simulink model "ad9361_rx_wlan_testbench_targeting_org"  (Simulink 10.0)
settings: Solver=FixedStepDiscrete  StartTime=0.0  StopTime=2  RelTol=1e-3
InitFcn:
  | % General
  | FFT = 64;
  | LSTFSymbol = FFT/4;
  | FS = 20e6;
  | 
  | % NCO
  | Fs = 20e6;
  | res = 0.05;
  | SFDR = 100;
  | N = ceil(log2(Fs/res));
  | %trueRes = Fs/(2^N);
  | %phaseInc = round(Fc*2^N/Fs);
  | QAB = round((SFDR-12)/6);
  | Dither = N - QAB;
  | 
  | %% LLTF
  | a = load('lltf.mat');
  | lltfFlip = conj(flipud(a.LLTF(:, 1)));
  | 
  | lltfFlip = lltfFlip./(max(abs(lltfFlip))) .* 2^0;
libraries: simulink x9, dsphdlfiltering x5, hdlsllib x4, commsource2 x1, dspmathops x1, dspsigops x1
(part 1 of 2)
settings Model: DataTypeOverride=Off  Creator=tcollins  LastModifiedBy=bhisma  SimulationMode=accelerator
settings Model: SuppressorTable=|
  | <?xml version="1.0" encoding="UTF-8" standalone="yes" ?>
  | <!DOCTYPE boost_serialization>
  | <boost_serialization signature="serialization::archive" version="15">
  | <DiagnosticSuppressor class_id="0" tracking_level="0" version="6">
  | 	<Table class_id="1" tracking_level="0" version="0">
  | 		<count>4</count>
  | 		<bucket_count>5</bucket_count>
  | 		<item_version>0</item_version>
  | 		<item class_id="2" tracking_level="0" version="0">
  | 			<first class_id="3" tracking_level="0" version="6">
  | 				<Source class_id="4" tracking_level="0" version="0">
  | 					<count>1</count>
  | 					<item_version>0</item_version>
  | 					<item>ad9361_rx_wlan_testbench_targeting_org/HDL_DUT/Control AGC/HDL Counter</item>
  | 				</Source>
  | 			</first>
  | 			<second class_id="5" tracking_level="0" version="6">
  | 				<SuppressedData class_id="6" tracking_level="0" version="0">
  | 					<count>2</count>
  | 					<bucket_count>2</bucket_count>
  | 					<item_version>0</item_version>
  | 					<item class_id="7" tracking_level="0" version="0">
  | 						<first class_id="8" tracking_level="0" version="6">
  | 							<ID>SimulinkFixedPoint:util:Overflowoccurred</ID>
  | 							<Cause>
  | 								<Source>
  | 									<count>0</count>
  | 									<item_version>0</item_version>
  | 								</Source>
  | 							</Cause>
  | 						</first>
  | 						<second class_id="9" tracking_level="0" version="6">
  | 							<Comment></Comment>
  | 							<User></User>
  | 							<LastModified class_id="10" tracking_level="0" version="0">
  | 								<ptime_date class_id="11" tracking_level="0" version="0">
  | 									<date>20160715</date>
  | 								</ptime_date>
  | 								<ptime_time_duration class_id="12" tracking_level="0" version="0">
  | 									<is_special>0</is_special>
  | 									<time_duration_hours>14</time_duration_hours>
  | 									<time_duration_minutes>21</time_duration_minutes>
  | 									<time_duration_seconds>36</time_duration_seconds>
  | 									<time_duration_fractional_seconds>0</time_duration_fractional_seconds>
  | 								</ptime_time_duration>
  | 							</LastModified>
  | 							<SuppressionType>1</SuppressionType>
  | 						</second>
  | 					</item>
  | 					<item>
  | 						<first>
  | 							<ID>Simulink:DataType:WarningOverFlowDetected</ID>
  | 							<Cause>
  | 								<Source>
  | 									<count>0</count>
  | 									<item_version>0</item_version>
  | 								</Source>
  | 							</Cause>
  | 						</first>
  | 						<second>
  | 							<Comment></Comment>
  | 							<User></User>
  | 							<LastModified>
  | 								<ptime_date>
  | 									<date>20160715</date>
  | 								</ptime_date>
  | 								<ptime_time_duration>
  | 									<is_special>0</is_special>
  | 									<time_duration_hours>14</time_duration_hours>
  | 									<time_duration_minutes>21</time_duration_minutes>
  | 									<time_duration_seconds>36</time_duration_seconds>
  | 									<time_duration_fractional_seconds>0</time_duration_fractional_seconds>
  | 								</ptime_time_duration>
  | 							</LastModified>
  | 							<SuppressionType>1</SuppressionType>
  | 						</second>
  | 					</item>
  | 				</SuppressedData>
  | 			</second>
  | 		</item>
  | 		<item>
  | 			<first>
  | 				<Source>
  | 					<count>1</count>
  | 					<item_version>0</item_version>
  | 					<item>ad9361_rx_wlan_testbench_targeting_org/HDL_DUT/Debug/HDL Counter3</item>
  | 				</Source>
  | 			</first>
  | 			<second>
  | 				<SuppressedData>
  | 					<count>2</count>
  | 					<bucket_count>2</bucket_count>
  | 					<item_version>0</item_version>
  | 					<item>
  | 						<first>
  | 							<ID>Simulink:DataType:WarningOverFlowDetected</ID>
  | 							<Cause>
  | 								<Source>
  | 									<count>0</count>
  | 									<item_version>0</item_version>
  | 								</Source>
  | 							</Cause>
  | 						</first>
  | 						<second>
  | 							<Comment></Comment>
  | 							<User></User>
  | 							<LastModified>
  | 								<ptime_date>
  | 									<date>20160715</date>
  | 								</ptime_date>
  | 								<ptime_time_duration>
  | 									<is_special>0</is_special>
  | 									<time_duration_hours>14</time_duration_hours>
  | 									<time_duration_minutes>21</time_duration_minutes>
  | 									<time_duration_seconds>36</time_duration_seconds>
  | 									<time_duration_fractional_seconds>0</time_duration_fractional_seconds>
  | 								</ptime_time_duration>
  | 							</LastModified>
  | 							<SuppressionType>1</SuppressionType>
  | 						</second>
  | 					</item>
  | 					<item>
  | 						<first>
  | 							<ID>SimulinkFixedPoint:util:Overflowoccurred</ID>
  | 							<Cause>
  | 								<Source>
  | 									<count>0</count>
  | 									<item_version>0</item_version>
  | 								</Source>
  | 							</Cause>
  | 						</first>
  | 						<second>
  | 							<Comment></Comment>
  | 							<User></User>
  | 							<LastModified>
  | 								<ptime_date>
  | 									<date>20160715</date>
  | 								</ptime_date>
  | 								<ptime_time_duration>
  | 									<is_special>0</is_special>
  | 									<time_duration_hours>14</time_duration_hours>
  | 									<time_duration_minutes>21</time_duration_minutes>
  | 									<time_duration_seconds>36</time_duration_seconds>
  | 									<time_duration_fractional_seconds>0</time_duration_fractional_seconds>
  | 								</ptime_time_duration>
  | 							</LastModified>
  | 							<SuppressionType>1</SuppressionType>
  | 						</second>
  | 					</item>
  | 				</SuppressedData>
  | 			</second>
  | 		</item>
  | 		<item>
  | 			<first>
  | 				<Source>
  | 					<count>1</count>
  | 					<item_version>0</item_version>
  | 					<item>ad9361_rx_wlan_testbench_targeting_org/HDL_DUT/Debug/HDL Counter2</item>
  | 				</Source>
  | 			</first>
  | 			<second>
  | 				<SuppressedData>
  | 					<count>2</count>
  | 					<bucket_count>2</bucket_count>
  | 					<item_version>0</item_version>
  | 					<item>
  | 						<first>
  | 							<ID>Simulink:DataType:WarningOverFlowDetected</ID>
  | 							<Cause>
  | 								<Source>
  | 									<count>0</count>
  | 									<item_version>0</item_version>
  | 								</Source>
  | 							</Cause>
  | 						</first>
  | 						<second>
  | 							<Comment></Comment>
  | 							<User></User>
  | 							<LastModified>
  | 								<ptime_date>
  | 									<date>20160715</date>
  | 								</ptime_date>
  | 								<ptime_time_duration>
  | 									<is_special>0</is_special>
  | 									<time_duration_hours>14</time_duration_hours>
  | 									<time_duration_minutes>21</time_duration_minutes>
  | 									<time_duration_seconds>36</time_duration_seconds>
  | 									<time_duration_fractional_seconds>0</time_duration_fractional_seconds>
  | 								</ptime_time_duration>
  | 							</LastModified>
  | 							<SuppressionType>1</SuppressionType>
  | 						</second>
  | 					</item>
  | 					<item>
  | 						<first>
  | 							<ID>SimulinkFixedPoint:util:Overflowoccurred</ID>
  | 							<Cause>
  | 								<Source>
  | 									<count>0</count>
  | 									<item_version>0</item_version>
  | 								</Source>
  | 							</Cause>
  | 						</first>
  | 						<second>
  | 							<Comment></Comment>
  | 							<User></User>
  | 							<LastModified>
  | 								<ptime_date>
  | 									<date>20160715</date>
  | 								</ptime_date>
  | 								<ptime_time_duration>
  | 									<is_special>0</is_special>
  | 									<time_duration_hours>14</time_duration_hours>
  | 									<time_duration_minutes>21</time_duration_minutes>
  | 									<time_duration_seconds>36</time_duration_seconds>
  | 									<time_duration_fractional_seconds>0</time_duration_fractional_seconds>
  | 								</ptime_time_duration>
  | 							</LastModified>
  | 							<SuppressionType>1</SuppressionType>
  | 						</second>
  | 					</item>
  | 				</SuppressedData>
  | 			</second>
  | 		</item>
  | 		<item>
  | 			<first>
  | 				<Source>
  | 					<count>1</count>
  | 					<item_version>0</item_version>
  | 					<item>ad9361_rx_wlan_testbench_targeting_org/HDL_DUT/Debug/HDL Counter1</item>
  | 				</Source>
  | 			</first>
  | 			<second>
  | 				<SuppressedData>
  | 					<count>2</count>
  | 					<bucket_count>2</bucket_count>
  | 					<item_version>0</item_version>
  | 					<item>
  | 						<first>
  | 							<ID>Simulink:DataType:WarningOverFlowDetected</ID>
  | 							<Cause>
  | 								<Source>
  | 									<count>0</count>
  | 									<item_version>0</item_version>
  | 								</Source>
  | 							</Cause>
  | 						</first>
  | 						<second>
  | 							<Comment></Comment>
  | 							<User></User>
  | 							<LastModified>
  | 								<ptime_date>
  | 									<date>20160715</date>
  | 								</ptime_date>
  | 								<ptime_time_duration>
  | 									<is_special>0</is_special>
  | 									<time_duration_hours>14</time_duration_hours>
  | 									<time_duration_minutes>21</time_duration_minutes>
  | 									<time_duration_seconds>36</time_duration_seconds>
  | 									<time_duration_fractional_seconds>0</time_duration_fractional_seconds>
  | 								</ptime_time_duration>
  | 							</LastModified>
  | 							<SuppressionType>1</SuppressionType>
  | 						</second>
  | 					</item>
  | 					<item>
  | 						<first>
  | 							<ID>SimulinkFixedPoint:util:Overflowoccurred</ID>
  | 							<Cause>
  | 								<Source>
  | 									<count>0</count>
  | 									<item_version>0</item_version>
  | 								</Source>
  | 							</Cause>
  | 						</first>
  | 						<second>
  | 							<Comment></Comment>
  | 							<User></User>
  | 							<LastModified>
  | 								<ptime_date>
  | 									<date>20160715</date>
  | 								</ptime_date>
  | 								<ptime_time_duration>
  | 									<is_special>0</is_special>
  | 									<time_duration_hours>14</time_duration_hours>
  | 									<time_duration_minutes>21</time_duration_minutes>
  | 									<time_duration_seconds>36</time_duration_seconds>
  | 									<time_duration_fractional_seconds>0</time_duration_fractional_seconds>
  | 								</ptime_time_duration>
  | 							</LastModified>
  | 							<SuppressionType>1</SuppressionType>
  | 						</second>
  | 					</item>
  | 				</SuppressedData>
  | 			</second>
  | 		</item>
  | 	</Table>
  | </DiagnosticSuppressor>
  | </boost_serialization>
settings DataIOCC: LimitDataPoints=on  SaveFormat=Dataset  SaveOutput=off  SaveTime=off
settings OptimizationCC: BlockReduction=off  ConditionallyExecuteInputs=off  DefaultParameterBehavior=Inlined
settings DebuggingCC: SignalRangeChecking=error  AlgebraicLoopMsg=error  UnderspecifiedInitializationDetection=Simplified  MergeDetectMultiDrivingBlocksExec=error  SingleTaskRateTransMsg=error  IntegerOverflowMsg=none  ParameterDowncastMsg=none  ParameterOverflowMsg=none  ParameterPrecisionLossMsg=none  AllowSymbolicDim=off  StrictBusMsg=ErrorOnBusTreatedAsVector  IntegerSaturationMsg=none
settings HardwareCC: ProdHWDeviceType=ASIC/FPGA->ASIC/FPGA  ProdEqTarget=off
settings ModelReferenceCC: PropagateSignalLabelsOutOfModel=on
settings GRTTargetCC: GeneratePreprocessorConditionals=Disable all  CombineOutputUpdateFcns=on  GRTInterface=off
settings ConfigComp: CovScope=ReferencedModels  CovExternalEMLEnable=off  CovSFcnEnable=off

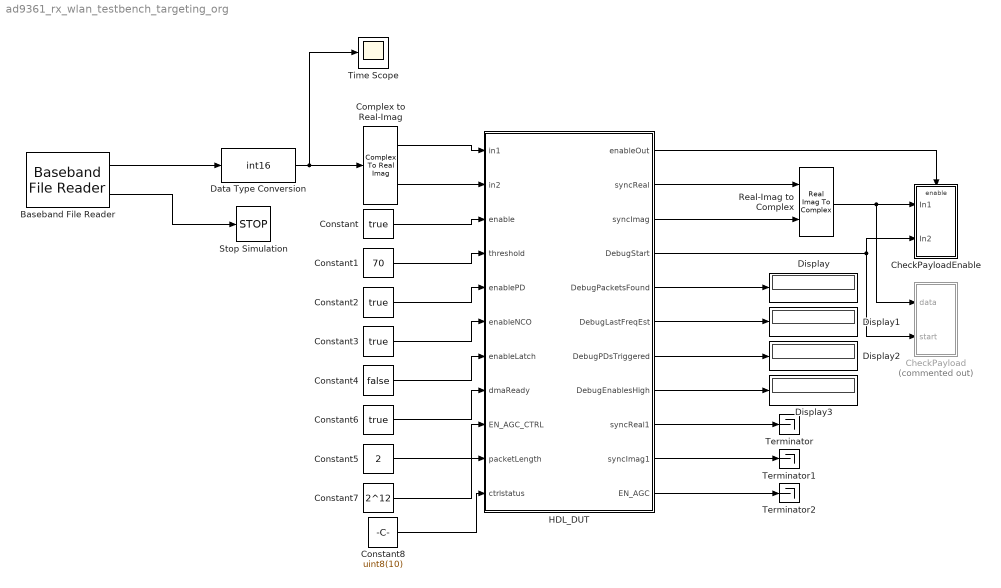
== system ad9361_rx_wlan_testbench_targeting_org ==
  Baseband File Reader : commsource2/Baseband File Reader  Filename=./captures/IQData_m25.bb  InheritSampleTimeFromFile=on  SampleTime=1  SamplesPerFrame=1  CyclicRepetition=off  FileEndOutputPort=on  SimulateUsing=Interpreted execution
      settings: SourceProductName=Communications Toolbox  SourceProductBaseCode=CM
  CheckPayload : Subsystem  Commented=on
  CheckPayloadEnable : Subsystem
  Complex to Real-Imag : ComplexToRealImag
  Constant{,2..3,6} (4 alike) : Constant  Value=true  SampleTime=-1
  Constant1 : Constant  Value=70  OutDataTypeStr=int16  SampleTime=-1
  Constant4 : Constant  Value=false  SampleTime=-1  LockScale=on
  Constant5 : Constant  Value=2  OutDataTypeStr=uint32  SampleTime=-1  LockScale=on
  Constant7 : Constant  Value=2^12  OutDataTypeStr=uint32  SampleTime=-1  LockScale=on
  Constant8 : Constant  Value=uint8(10)  OutDataTypeStr=uint8  SampleTime=-1  LockScale=on
  Data Type Conversion : DataTypeConversion  OutDataTypeStr=int16
  Display{,1..3} (4 alike) : Display
  HDL_DUT : Subsystem  TreatAsAtomicUnit=on
  Real-Imag to Complex : RealImagToComplex
  Stop Simulation : Stop
  Terminator : Terminator
  Terminator1 : Terminator
  Terminator2 : Terminator
  Time Scope : Scope
  wires:
  Constant/1 -> HDL_DUT/3(enable)
  Complex to Real-Imag/1 -> HDL_DUT/1(in1)
  Complex to Real-Imag/2 -> HDL_DUT/2(in2)
  Baseband File Reader/1 -> Data Type Conversion/1
  Constant1/1 -> HDL_DUT/4(threshold)
  Constant2/1 -> HDL_DUT/5(enablePD)
  Constant3/1 -> HDL_DUT/6(enableNCO)
  HDL_DUT/7(DebugPDsTriggered) -> Display2/1
  HDL_DUT/5(DebugPacketsFound) -> Display/1
  Real-Imag to Complex/1 -> CheckPayload/1(data), CheckPayloadEnable/1(In1)
  HDL_DUT/4(DebugStart) -> CheckPayloadEnable/2(In2), CheckPayload/2(start)
  HDL_DUT/6(DebugLastFreqEst) -> Display1/1
  HDL_DUT/8(DebugEnablesHigh) -> Display3/1
  HDL_DUT/2(syncReal) -> Real-Imag to Complex/1
  HDL_DUT/3(syncImag) -> Real-Imag to Complex/2
  HDL_DUT/1(enableOut) -> CheckPayloadEnable/Enable
  Data Type Conversion/1 -> Time Scope/1, Complex to Real-Imag/1
  HDL_DUT/9(syncReal1) -> Terminator/1
  HDL_DUT/10(syncImag1) -> Terminator1/1
  Constant4/1 -> HDL_DUT/7(enableLatch)
  Constant5/1 -> HDL_DUT/9(EN_AGC_CTRL)
  Constant6/1 -> HDL_DUT/8(dmaReady)
  Constant7/1 -> HDL_DUT/10(packetLength)
  HDL_DUT/11(EN_AGC) -> Terminator2/1
  Baseband File Reader/2 -> Stop Simulation/1
  Constant8/1 -> HDL_DUT/11(ctrlstatus)

== system ad9361_rx_wlan_testbench_targeting_org/CheckPayload ==
  data : Inport  OutDataTypeStr=int16
  start : Inport  Port=2
  Check LSIG1 : MATLAB Function  TreatAsAtomicUnit=on
  SaveData : Subsystem
  wires:
  Check LSIG1/2(goodPackets) -> SaveData/1(In1)
  start/1 -> Check LSIG1/1(start)
  Check LSIG1/1(valid) -> SaveData/Enable
  data/1 -> Check LSIG1/2(data)
  Check LSIG1/3(badPackets) -> SaveData/2(In2)

== system ad9361_rx_wlan_testbench_targeting_org/CheckPayloadEnable ==
  In1 : Inport
  In2 : Inport  Port=2
  Enable : EnablePort
  Check LSIG1 : MATLAB Function  TreatAsAtomicUnit=on
  SaveData : Subsystem
  wires:
  Check LSIG1/2(goodPackets) -> SaveData/1(In1)
  Check LSIG1/1(valid) -> SaveData/Enable
  In1/1 -> Check LSIG1/2(data)
  Check LSIG1/3(badPackets) -> SaveData/2(In2)
  In2/1 -> Check LSIG1/1(start)

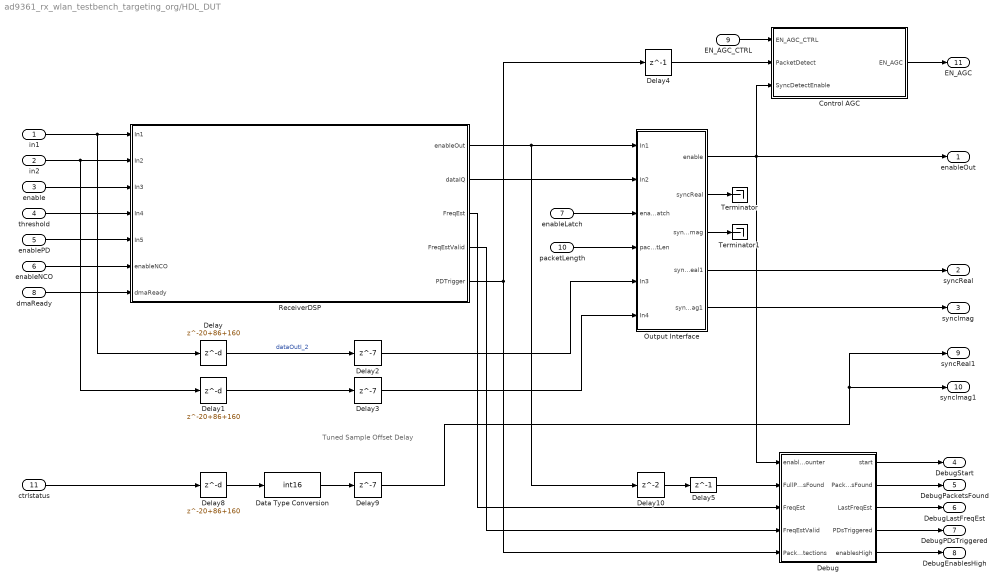
== system ad9361_rx_wlan_testbench_targeting_org/HDL_DUT ==
  note: Tuned Sample Offset Delay
  in1 : Inport  OutDataTypeStr=int16
  in2 : Inport  Port=2  OutDataTypeStr=int16
  enable : Inport  Port=3  OutDataTypeStr=boolean  LockScale=on
  threshold : Inport  Port=4  OutDataTypeStr=int16  LockScale=on
  enablePD : Inport  Port=5  OutDataTypeStr=boolean  LockScale=on
  enableNCO : Inport  Port=6  OutDataTypeStr=boolean  LockScale=on
  enableLatch : Inport  Port=7  OutDataTypeStr=boolean  LockScale=on
  dmaReady : Inport  Port=8  OutDataTypeStr=boolean
  EN_AGC_CTRL : Inport  Port=9  OutDataTypeStr=uint32
  packetLength : Inport  Port=10  OutDataTypeStr=uint32  LockScale=on
  ctrlstatus : Inport  Port=11  OutDataTypeStr=uint8
  Control AGC : Subsystem
  Data Type Conversion : DataTypeConversion  OutDataTypeStr=int16
  Debug : Subsystem
  Delay : Delay  DelayLength=20+86+160
  Delay1 : Delay  DelayLength=20+86+160
  Delay10 : Delay
  Delay2 : Delay  DelayLength=7
  Delay3 : Delay  DelayLength=7
  Delay4 : Delay  DelayLength=1
  Delay5 : Delay  DelayLength=1
  Delay8 : Delay  DelayLength=20+86+160
  Delay9 : Delay  DelayLength=7
  Output Interface : Subsystem
  ReceiverDSP : Subsystem
  Terminator : Terminator
  Terminator1 : Terminator
  enableOut : Outport  VectorParamsAs1DForOutWhenUnconnected=off
  syncReal : Outport  Port=2  OutDataTypeStr=int16  VectorParamsAs1DForOutWhenUnconnected=off
  syncImag : Outport  Port=3  OutDataTypeStr=int16  VectorParamsAs1DForOutWhenUnconnected=off
  DebugStart : Outport  Port=4  VectorParamsAs1DForOutWhenUnconnected=off
  DebugPacketsFound : Outport  Port=5  VectorParamsAs1DForOutWhenUnconnected=off
  DebugLastFreqEst : Outport  Port=6  VectorParamsAs1DForOutWhenUnconnected=off
  DebugPDsTriggered : Outport  Port=7  VectorParamsAs1DForOutWhenUnconnected=off
  DebugEnablesHigh : Outport  Port=8  VectorParamsAs1DForOutWhenUnconnected=off
  syncReal1 : Outport  Port=9  OutDataTypeStr=int16  VectorParamsAs1DForOutWhenUnconnected=off
  syncImag1 : Outport  Port=10  OutDataTypeStr=int16  VectorParamsAs1DForOutWhenUnconnected=off
  EN_AGC : Outport  Port=11  OutDataTypeStr=boolean  VectorParamsAs1DForOutWhenUnconnected=off
  wires:
  Debug/2(PacketsFound) -> DebugPacketsFound/1
  Debug/3(LastFreqEst) -> DebugLastFreqEst/1
  Debug/5(enablesHigh) -> DebugEnablesHigh/1
  Debug/4(PDsTriggered) -> DebugPDsTriggered/1
  Debug/1(start) -> DebugStart/1
  Output Interface/1(enable) -> enableOut/1, Control AGC/3(SyncDetectEnable), Debug/1(enableCounter)
  ReceiverDSP/1(enableOut) -> Output Interface/1(In1), Delay10/1
  in2/1 -> Delay1/1, ReceiverDSP/2(In2)
  enable/1 -> ReceiverDSP/3(In3)
  threshold/1 -> ReceiverDSP/4(In4)
  enablePD/1 -> ReceiverDSP/5(In5)
  enableNCO/1 -> ReceiverDSP/6(enableNCO)
  ReceiverDSP/3(FreqEst) -> Debug/3(FreqEst)
  ReceiverDSP/4(FreqEstValid) -> Debug/4(FreqEstValid)
  ReceiverDSP/5(PDTrigger) -> Delay4/1, Debug/5(PacketDetections)
  in1/1 -> Delay/1, ReceiverDSP/1(In1)
  Delay/1 -> Delay2/1  "dataOutI_2"
  enableLatch/1 -> Output Interface/3(enableLatch)
  Control AGC/1(EN_AGC) -> EN_AGC/1
  EN_AGC_CTRL/1 -> Control AGC/1(EN_AGC_CTRL)
  dmaReady/1 -> ReceiverDSP/7(dmaReady)
  Output Interface/2(syncReal) -> Terminator/1
  Output Interface/3(syncImag) -> Terminator1/1
  Delay1/1 -> Delay3/1
  packetLength/1 -> Output Interface/4(packetLen)
  Delay4/1 -> Control AGC/2(PacketDetect)
  Delay5/1 -> Debug/2(FullPacketsFound)
  ReceiverDSP/2(dataIQ) -> Output Interface/2(In2)
  Delay10/1 -> Delay5/1
  Output Interface/4(syncReal1) -> syncReal/1
  Output Interface/5(syncImag1) -> syncImag/1
  Delay2/1 -> Output Interface/5(In3)
  Delay3/1 -> Output Interface/6(In4)
  ctrlstatus/1 -> Delay8/1
  Delay8/1 -> Data Type Conversion/1
  Delay9/1 -> syncImag1/1, syncReal1/1
  Data Type Conversion/1 -> Delay9/1

== system ad9361_rx_wlan_testbench_targeting_org/CheckPayload/SaveData ==
  In1 : Inport
  In2 : Inport  Port=2
  Enable : EnablePort
  To Workspace : ToWorkspace  VariableName=goodpackets  SampleTime=-1
      settings: Save2DSignal=2-D array (concatenate along first dimension)
  To Workspace1 : ToWorkspace  VariableName=badpackets  SampleTime=-1
      settings: Save2DSignal=2-D array (concatenate along first dimension)
  wires:
  In1/1 -> To Workspace/1
  In2/1 -> To Workspace1/1

== system ad9361_rx_wlan_testbench_targeting_org/CheckPayloadEnable/SaveData ==
  In1 : Inport
  In2 : Inport  Port=2
  Enable : EnablePort
  To Workspace : ToWorkspace  VariableName=goodpackets  SampleTime=-1
      settings: Save2DSignal=2-D array (concatenate along first dimension)
  To Workspace1 : ToWorkspace  VariableName=badpackets  SampleTime=-1
      settings: Save2DSignal=2-D array (concatenate along first dimension)
  wires:
  In1/1 -> To Workspace/1
  In2/1 -> To Workspace1/1

== system ad9361_rx_wlan_testbench_targeting_org/HDL_DUT/Control AGC ==
  note: EN_AGC signal should be low during packet so it says in lock state
  EN_AGC_CTRL : Inport
  PacketDetect : Inport  Port=2
  SyncDetectEnable : Inport  Port=3
  Compare To Constant : simulink/Logic and Bit Operations/Compare To Constant  relop=<=  const=20+86+160+40  OutDataTypeStr=boolean
  Constant : Constant  Value=false  SampleTime=-1
  Constant1 : Constant  Value=true  SampleTime=-1
  HDL Counter : hdlsllib/Sources/HDL Counter  CountType=Count limited  CountInit=0  CountStep=1  CountMax=1023  CountFromType=Initial value  CountFrom=0  CountResetPort=on  CountLoadPort=off  CountEnbPort=on  CountDirPort=off  CountDataType=Unsigned  CountWordLen=16  CountFracLen=0  CountSampTime=1
      settings: SourceProductBaseCode=HD
  Index Vector : MultiPortSwitch  DataPortOrder=Zero-based contiguous  zeroidx=on
  Logical Operator : Logic  Operator=NOT  AllPortsSameDT=off  OutDataTypeStr=boolean
  OR : Logic  Operator=OR  IconShape=distinctive  AllPortsSameDT=off  OutDataTypeStr=boolean
  EN_AGC : Outport  VectorParamsAs1DForOutWhenUnconnected=off
  wires:
  PacketDetect/1 -> HDL Counter/1
  HDL Counter/1 -> Compare To Constant/1
  Compare To Constant/1 -> OR/1, HDL Counter/2
  SyncDetectEnable/1 -> OR/2
  OR/1 -> Index Vector/4
  Index Vector/1 -> Logical Operator/1
  EN_AGC_CTRL/1 -> Index Vector/1
  Constant/1 -> Index Vector/2
  Constant1/1 -> Index Vector/3
  Logical Operator/1 -> EN_AGC/1

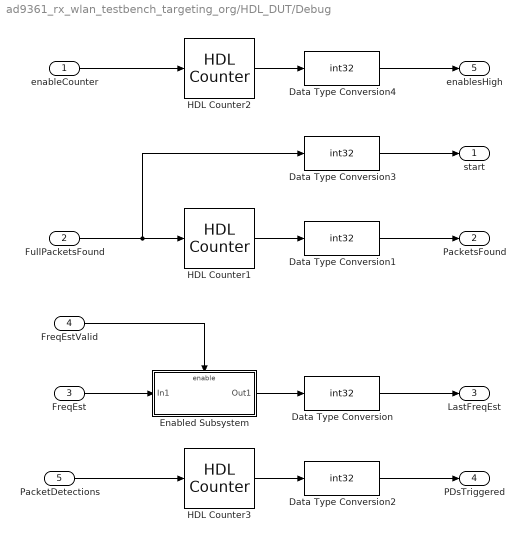
== system ad9361_rx_wlan_testbench_targeting_org/HDL_DUT/Debug ==
  enableCounter : Inport
  FullPacketsFound : Inport  Port=2
  FreqEst : Inport  Port=3  OutDataTypeStr=fixdt(1,11,-3)
  FreqEstValid : Inport  Port=4
  PacketDetections : Inport  Port=5
  Data Type Conversion{,1..4} (5 alike) : DataTypeConversion  OutDataTypeStr=int32
  Enabled Subsystem : Subsystem  TreatAsAtomicUnit=on
  HDL Counter1 : hdlsllib/Sources/HDL Counter  CountType=Count limited  CountInit=0  CountStep=1  CountMax=2^31-1  CountFromType=Initial value  CountFrom=0  CountResetPort=off  CountLoadPort=off  CountEnbPort=on  CountDirPort=off  CountDataType=Unsigned  CountWordLen=31  CountFracLen=0  CountSampTime=1
      settings: SourceProductBaseCode=HD
  HDL Counter2 : hdlsllib/Sources/HDL Counter  CountType=Count limited  CountInit=0  CountStep=1  CountMax=2^31-1  CountFromType=Initial value  CountFrom=0  CountResetPort=off  CountLoadPort=off  CountEnbPort=on  CountDirPort=off  CountDataType=Unsigned  CountWordLen=31  CountFracLen=0  CountSampTime=1
      settings: SourceProductBaseCode=HD
  HDL Counter3 : hdlsllib/Sources/HDL Counter  CountType=Count limited  CountInit=0  CountStep=1  CountMax=2^31-1  CountFromType=Initial value  CountFrom=0  CountResetPort=off  CountLoadPort=off  CountEnbPort=on  CountDirPort=off  CountDataType=Unsigned  CountWordLen=31  CountFracLen=0  CountSampTime=1
      settings: SourceProductBaseCode=HD
  start : Outport  VectorParamsAs1DForOutWhenUnconnected=off
  PacketsFound : Outport  Port=2  VectorParamsAs1DForOutWhenUnconnected=off
  LastFreqEst : Outport  Port=3  VectorParamsAs1DForOutWhenUnconnected=off
  PDsTriggered : Outport  Port=4  VectorParamsAs1DForOutWhenUnconnected=off
  enablesHigh : Outport  Port=5  VectorParamsAs1DForOutWhenUnconnected=off
  wires:
  FullPacketsFound/1 -> HDL Counter1/1, Data Type Conversion3/1
  HDL Counter1/1 -> Data Type Conversion1/1
  FreqEst/1 -> Enabled Subsystem/1(In1)
  FreqEstValid/1 -> Enabled Subsystem/Enable
  Enabled Subsystem/1(Out1) -> Data Type Conversion/1
  Data Type Conversion/1 -> LastFreqEst/1
  Data Type Conversion1/1 -> PacketsFound/1
  HDL Counter3/1 -> Data Type Conversion2/1
  Data Type Conversion2/1 -> PDsTriggered/1
  PacketDetections/1 -> HDL Counter3/1
  Data Type Conversion3/1 -> start/1
  Data Type Conversion4/1 -> enablesHigh/1
  HDL Counter2/1 -> Data Type Conversion4/1
  enableCounter/1 -> HDL Counter2/1

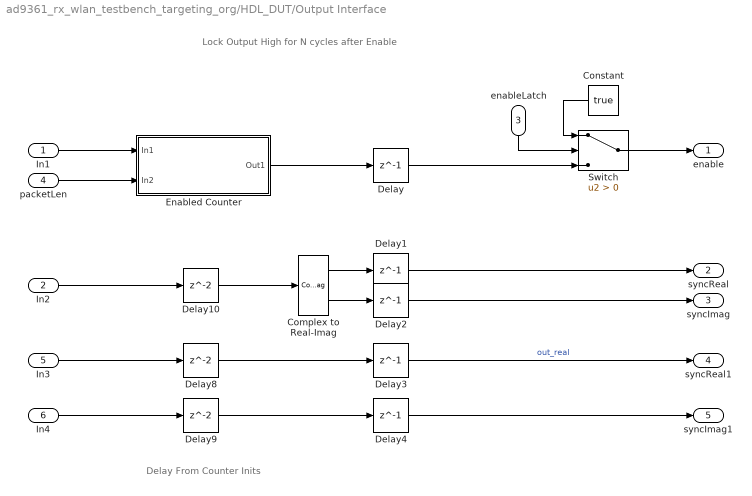
== system ad9361_rx_wlan_testbench_targeting_org/HDL_DUT/Output Interface ==
  note: Delay From Counter Inits
  note: Lock Output High for N cycles after Enable
  In1 : Inport
  In2 : Inport  Port=2  OutDataTypeStr=fixdt(1,11,-1)
  enableLatch : Inport  Port=3
  packetLen : Inport  Port=4
  In3 : Inport  Port=5
  In4 : Inport  Port=6
  Complex to Real-Imag : ComplexToRealImag
  Constant : Constant  Value=true  SampleTime=-1
  Delay{,1..4} (5 alike) : Delay  DelayLength=1
  Delay10 : Delay
  Delay8 : Delay
  Delay9 : Delay
  Enabled Counter : Subsystem
  Switch : Switch  Criteria=u2 > Threshold
  enable : Outport  VectorParamsAs1DForOutWhenUnconnected=off
  syncReal : Outport  Port=2  VectorParamsAs1DForOutWhenUnconnected=off
  syncImag : Outport  Port=3  VectorParamsAs1DForOutWhenUnconnected=off
  syncReal1 : Outport  Port=4  VectorParamsAs1DForOutWhenUnconnected=off
  syncImag1 : Outport  Port=5  VectorParamsAs1DForOutWhenUnconnected=off
  wires:
  In2/1 -> Delay10/1
  In1/1 -> Enabled Counter/1(In1)
  Constant/1 -> Switch/1
  enableLatch/1 -> Switch/2
  packetLen/1 -> Enabled Counter/2(In2)
  Complex to Real-Imag/1 -> Delay1/1
  Complex to Real-Imag/2 -> Delay2/1
  Switch/1 -> enable/1
  Delay/1 -> Switch/3
  Delay1/1 -> syncReal/1
  Delay2/1 -> syncImag/1
  Enabled Counter/1(Out1) -> Delay/1
  Delay10/1 -> Complex to Real-Imag/1
  Delay9/1 -> Delay4/1
  Delay8/1 -> Delay3/1
  In4/1 -> Delay9/1
  In3/1 -> Delay8/1
  Delay3/1 -> syncReal1/1  "out_real"
  Delay4/1 -> syncImag1/1

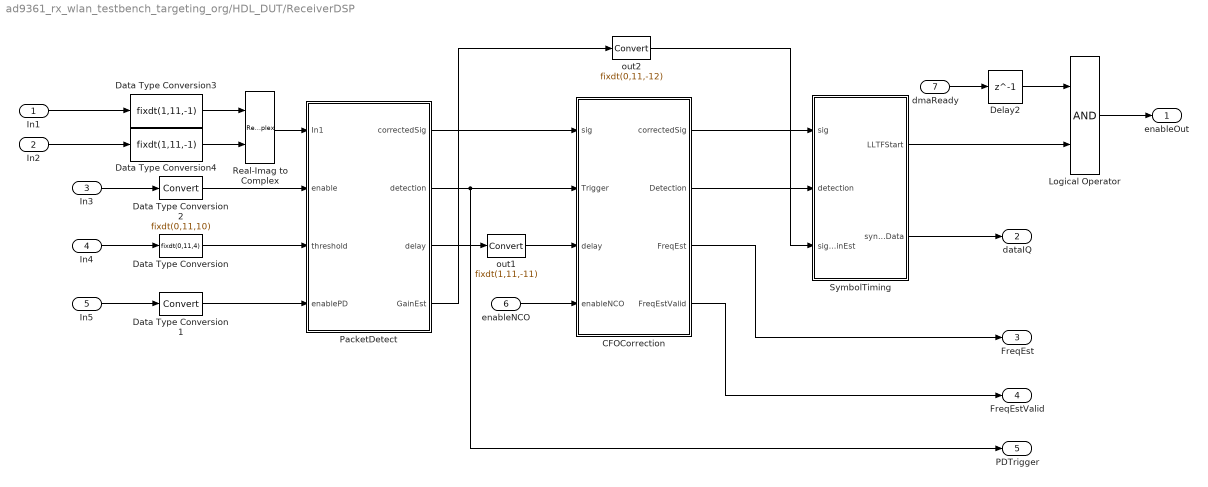
== system ad9361_rx_wlan_testbench_targeting_org/HDL_DUT/ReceiverDSP ==
  In1 : Inport  OutDataTypeStr=int16
  In2 : Inport  Port=2  OutDataTypeStr=int16
  In3 : Inport  Port=3
  In4 : Inport  Port=4
  In5 : Inport  Port=5
  enableNCO : Inport  Port=6  OutDataTypeStr=boolean  LockScale=on
  dmaReady : Inport  Port=7
  CFOCorrection : Subsystem
  Data Type Conversion : DataTypeConversion  OutDataTypeStr=fixdt(0,11,4)
  Data Type Conversion1 : DataTypeConversion
  Data Type Conversion2 : DataTypeConversion  OutDataTypeStr=fixdt(0,11,10)
  Data Type Conversion3 : DataTypeConversion  OutDataTypeStr=fixdt(1,11,-1)
  Data Type Conversion4 : DataTypeConversion  OutDataTypeStr=fixdt(1,11,-1)
  Delay2 : Delay  DelayLength=1
  Logical Operator : Logic  AllPortsSameDT=off  OutDataTypeStr=boolean
  PacketDetect : Subsystem
  Real-Imag to Complex : RealImagToComplex
  SymbolTiming : Subsystem
  out1 : DataTypeConversion  OutDataTypeStr=fixdt(1,11,-11)
  out2 : DataTypeConversion  OutDataTypeStr=fixdt(0,11,-12)
  enableOut : Outport  VectorParamsAs1DForOutWhenUnconnected=off
  dataIQ : Outport  Port=2  OutDataTypeStr=fixdt(1,11,-1)  VectorParamsAs1DForOutWhenUnconnected=off
  FreqEst : Outport  Port=3  OutDataTypeStr=fixdt(1,11,-3)  VectorParamsAs1DForOutWhenUnconnected=off
  FreqEstValid : Outport  Port=4  VectorParamsAs1DForOutWhenUnconnected=off
  PDTrigger : Outport  Port=5  VectorParamsAs1DForOutWhenUnconnected=off
  wires:
  PacketDetect/1(correctedSig) -> CFOCorrection/1(sig)
  In2/1 -> Data Type Conversion4/1
  CFOCorrection/3(FreqEst) -> FreqEst/1
  Data Type Conversion/1 -> PacketDetect/3(threshold)
  out2/1 -> SymbolTiming/3(sigGainEst)
  In5/1 -> Data Type Conversion1/1
  In3/1 -> Data Type Conversion2/1
  Data Type Conversion2/1 -> PacketDetect/2(enable)
  PacketDetect/3(delay) -> out1/1
  SymbolTiming/2(syncedData) -> dataIQ/1
  Real-Imag to Complex/1 -> PacketDetect/1(In1)
  CFOCorrection/2(Detection) -> SymbolTiming/2(detection)
  out1/1 -> CFOCorrection/3(delay)
  In4/1 -> Data Type Conversion/1
  CFOCorrection/1(correctedSig) -> SymbolTiming/1(sig)
  PacketDetect/4(GainEst) -> out2/1
  PacketDetect/2(detection) -> PDTrigger/1, CFOCorrection/2(Trigger)
  enableNCO/1 -> CFOCorrection/4(enableNCO)
  CFOCorrection/4(FreqEstValid) -> FreqEstValid/1
  Data Type Conversion1/1 -> PacketDetect/4(enablePD)
  In1/1 -> Data Type Conversion3/1
  Data Type Conversion3/1 -> Real-Imag to Complex/1
  Data Type Conversion4/1 -> Real-Imag to Complex/2
  SymbolTiming/1(LLTFStart) -> Logical Operator/2
  Logical Operator/1 -> enableOut/1
  dmaReady/1 -> Delay2/1
  Delay2/1 -> Logical Operator/1

== system ad9361_rx_wlan_testbench_targeting_org/HDL_DUT/Debug/Enabled Subsystem ==
  In1 : Inport  OutDataTypeStr=fixdt(1,11,-3)
  Enable : EnablePort
  Delay : Delay  DelayLength=1
  Out1 : Outport  OutDataTypeStr=fixdt(1,11,-3)  InitialOutput=false  VectorParamsAs1DForOutWhenUnconnected=off
  wires:
  In1/1 -> Delay/1
  Delay/1 -> Out1/1

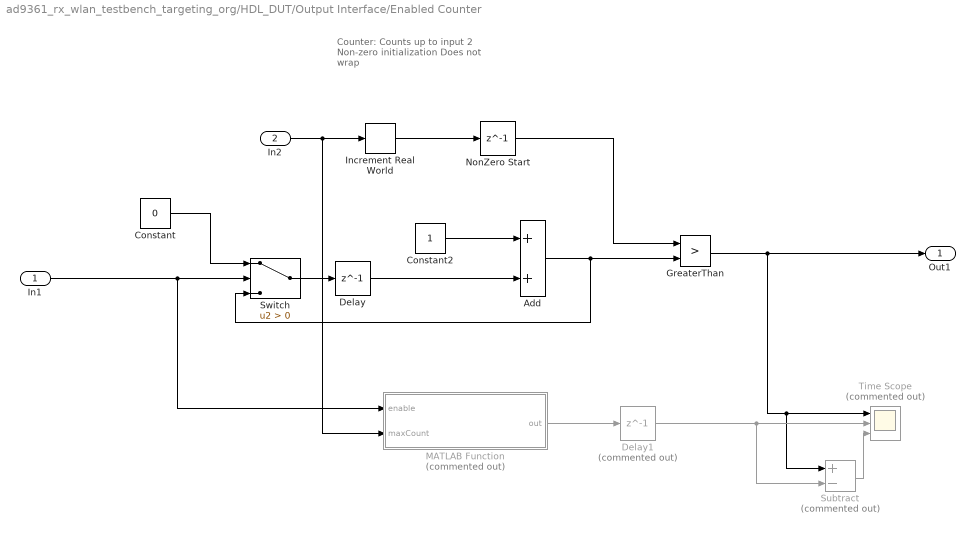
== system ad9361_rx_wlan_testbench_targeting_org/HDL_DUT/Output Interface/Enabled Counter ==
  note: Counter:
      | Counts up to input 2
      | Non-zero initialization
      | Does not wrap
  In1 : Inport
  In2 : Inport  Port=2
  Add : Sum  AccumDataTypeStr=uint16  OutDataTypeStr=uint16  SaturateOnIntegerOverflow=on
  Constant : Constant  Value=0  OutDataTypeStr=uint16  SampleTime=-1
  Constant2 : Constant  OutDataTypeStr=uint8  SampleTime=-1
  Delay : Delay  DelayLength=1  InitialCondition=2^15
  Delay1 : Delay  Commented=on  DelayLength=1
  GreaterThan : RelationalOperator  Operator=>  OutDataTypeStr=boolean  RndMeth=Simplest
  Increment Real World : simulink/Additional Math & Discrete/Additional Math: Increment - Decrement/Increment Real World
      settings: SourceProductName=Simulink  SourceProductBaseCode=SL
  MATLAB Function : MATLAB Function  Commented=on  TreatAsAtomicUnit=on
  NonZero Start : Delay  DelayLength=1  InitialCondition=2^14
  Subtract : Sum  Commented=on  Inputs=+-
  Switch : Switch  Criteria=u2 > Threshold
  Time Scope : Scope  Commented=on  NumInputPorts=3
  Out1 : Outport  VectorParamsAs1DForOutWhenUnconnected=off
  wires:
  Add/1 -> Switch/3, GreaterThan/2
  GreaterThan/1 -> Out1/1, Subtract/1, Time Scope/1
  NonZero Start/1 -> GreaterThan/1
  Constant2/1 -> Add/1
  Increment Real World/1 -> NonZero Start/1
  In2/1 -> MATLAB Function/2(maxCount), Increment Real World/1
  Delay/1 -> Add/2
  Switch/1 -> Delay/1
  In1/1 -> MATLAB Function/1(enable), Switch/2
  Constant/1 -> Switch/1
  MATLAB Function/1(out) -> Delay1/1
  Subtract/1 -> Time Scope/3
  Delay1/1 -> Subtract/2, Time Scope/2

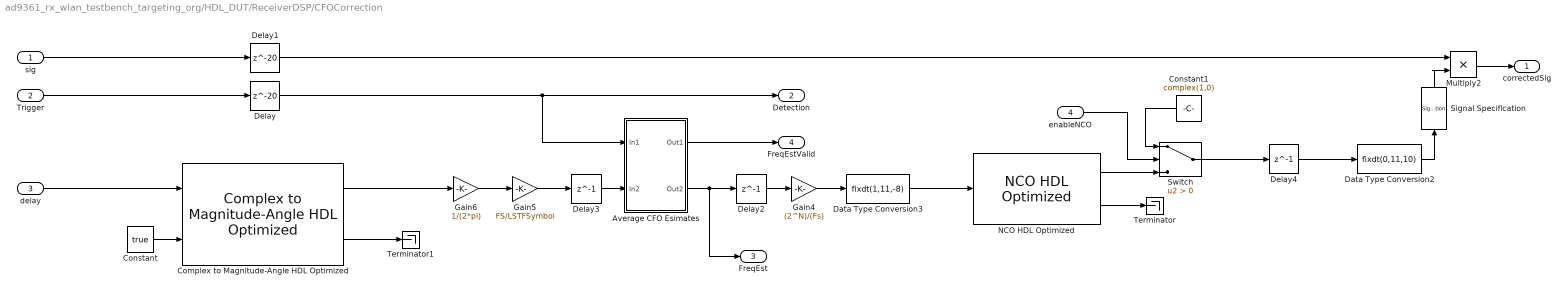
== system ad9361_rx_wlan_testbench_targeting_org/HDL_DUT/ReceiverDSP/CFOCorrection ==
  sig : Inport  OutDataTypeStr=fixdt(1,11,-1)
  Trigger : Inport  Port=2
  delay : Inport  Port=3  OutDataTypeStr=fixdt(1,11,-11)
  enableNCO : Inport  Port=4  OutDataTypeStr=boolean
  Average CFO Esimates : Subsystem
  Complex to Magnitude-Angle HDL Optimized : dspmathops/Complex to Magnitude-Angle HDL Optimized  NumIterationsSource=Auto  NumIterations=10  OutputFormat=Angle  AngleFormat=Radians  ScaleOutput=on  SimulateUsing=Code generation
      settings: SourceProductName=DSP System Toolbox  SourceProductBaseCode=DS
  Constant : Constant  Value=true  OutDataTypeStr=boolean  SampleTime=-1
  Constant1 : Constant  Value=complex(1,0)  OutDataTypeStr=fixdt(0,11,10)  SampleTime=-1
  Data Type Conversion2 : DataTypeConversion  OutDataTypeStr=fixdt(0,11,10)
  Data Type Conversion3 : DataTypeConversion  OutDataTypeStr=fixdt(1,11,-8)
  Delay : Delay  DelayLength=20
  Delay1 : Delay  DelayLength=20
  Delay2 : Delay  DelayLength=1
  Delay3 : Delay  DelayLength=1
  Delay4 : Delay  DelayLength=1
  Gain4 : Gain  Gain=(2^N)/(Fs)  ParamDataTypeStr=fixdt(0,11,6)  OutDataTypeStr=fixdt(1,11,-8)
  Gain5 : Gain  Gain=FS/LSTFSymbol  ParamDataTypeStr=fixdt(0,11,-10)  OutDataTypeStr=fixdt(1,11,-10)
  Gain6 : Gain  Gain=1/(2*pi)  ParamDataTypeStr=fixdt(0,11,13)  OutDataTypeStr=fixdt(1,11,10)
  Multiply2 : Product  OutDataTypeStr=fixdt(1,11,-1)
  NCO HDL Optimized : dspsigops/NCO HDL Optimized  PhaseIncrementSource=Input port  PhaseIncrement=100  PhaseOffsetSource=Property  PhaseOffset=0  DitherSource=Property  NumDitherBits=Dither  PhaseQuantization=on  NumQuantizerAccumulatorBits=QAB  LUTCompress=off  ResetAction=off  ValidInputPort=off  Waveform=Complex exponential  PhasePort=off  SimulateUsing=Code generation  AccumulatorWL=N  OutputDataType=Binary point scaling  OutputWL=N  OutputFL=N-1
      settings: SourceProductName=DSP System Toolbox  SourceProductBaseCode=DS
  Signal Specification : SignalSpecification  OutDataTypeStr=fixdt(0,11,10)  Dimensions=1
  Switch : Switch  Criteria=u2 > Threshold  OutDataTypeStr=fixdt(0,11,10)
  Terminator : Terminator
  Terminator1 : Terminator
  correctedSig : Outport  OutDataTypeStr=fixdt(1,11,-1)  VectorParamsAs1DForOutWhenUnconnected=off
  Detection : Outport  Port=2  VectorParamsAs1DForOutWhenUnconnected=off
  FreqEst : Outport  Port=3  OutDataTypeStr=fixdt(1,11,-3)  VectorParamsAs1DForOutWhenUnconnected=off
  FreqEstValid : Outport  Port=4  VectorParamsAs1DForOutWhenUnconnected=off
  wires:
  sig/1 -> Delay1/1
  Multiply2/1 -> correctedSig/1
  Data Type Conversion2/1 -> Signal Specification/1
  Gain4/1 -> Data Type Conversion3/1
  NCO HDL Optimized/2 -> Terminator/1
  Constant/1 -> Complex to Magnitude-Angle HDL Optimized/2
  Gain6/1 -> Gain5/1
  Complex to Magnitude-Angle HDL Optimized/2 -> Terminator1/1
  Trigger/1 -> Delay/1
  Complex to Magnitude-Angle HDL Optimized/1 -> Gain6/1
  Average CFO Esimates/2(Out2) -> FreqEst/1, Delay2/1
  Gain5/1 -> Delay3/1
  Average CFO Esimates/1(Out1) -> FreqEstValid/1
  delay/1 -> Complex to Magnitude-Angle HDL Optimized/1
  Delay/1 -> Average CFO Esimates/1(In1), Detection/1
  Delay1/1 -> Multiply2/1
  Data Type Conversion3/1 -> NCO HDL Optimized/1
  Constant1/1 -> Switch/1
  enableNCO/1 -> Switch/2
  NCO HDL Optimized/1 -> Switch/3
  Switch/1 -> Delay4/1
  Signal Specification/1 -> Multiply2/2
  Delay2/1 -> Gain4/1
  Delay3/1 -> Average CFO Esimates/2(In2)
  Delay4/1 -> Data Type Conversion2/1

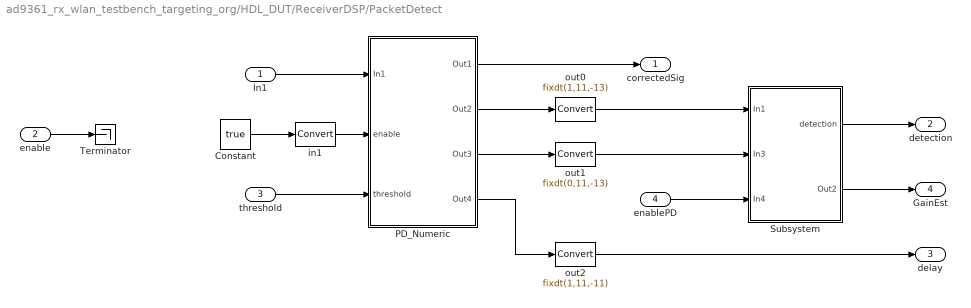
== system ad9361_rx_wlan_testbench_targeting_org/HDL_DUT/ReceiverDSP/PacketDetect ==
  In1 : Inport  OutDataTypeStr=fixdt(1,11,-1)
  enable : Inport  Port=2  OutDataTypeStr=fixdt(0,11,10)
  threshold : Inport  Port=3  OutDataTypeStr=fixdt(0,11,4)
  enablePD : Inport  Port=4  OutDataTypeStr=boolean
  Constant : Constant  Value=true  SampleTime=-1
  PD_Numeric : Subsystem
  Subsystem : Subsystem
  Terminator : Terminator
  in1 : DataTypeConversion
  out0 : DataTypeConversion  OutDataTypeStr=fixdt(1,11,-13)  SaturateOnIntegerOverflow=on
  out1 : DataTypeConversion  OutDataTypeStr=fixdt(0,11,-13)
  out2 : DataTypeConversion  OutDataTypeStr=fixdt(1,11,-11)
  correctedSig : Outport  OutDataTypeStr=fixdt(1,11,-1)  VectorParamsAs1DForOutWhenUnconnected=off
  detection : Outport  Port=2  VectorParamsAs1DForOutWhenUnconnected=off
  delay : Outport  Port=3  OutDataTypeStr=fixdt(1,11,-11)  VectorParamsAs1DForOutWhenUnconnected=off
  GainEst : Outport  Port=4  OutDataTypeStr=fixdt(0,11,-12)  VectorParamsAs1DForOutWhenUnconnected=off
  wires:
  PD_Numeric/3(Out3) -> out1/1
  PD_Numeric/1(Out1) -> correctedSig/1
  PD_Numeric/2(Out2) -> out0/1
  PD_Numeric/4(Out4) -> out2/1
  In1/1 -> PD_Numeric/1(In1)
  in1/1 -> PD_Numeric/2(enable)
  out2/1 -> delay/1
  threshold/1 -> PD_Numeric/3(threshold)
  Subsystem/2(Out2) -> GainEst/1
  out0/1 -> Subsystem/1(In1)
  out1/1 -> Subsystem/2(In3)
  enablePD/1 -> Subsystem/3(In4)
  Subsystem/1(detection) -> detection/1
  Constant/1 -> in1/1
  enable/1 -> Terminator/1

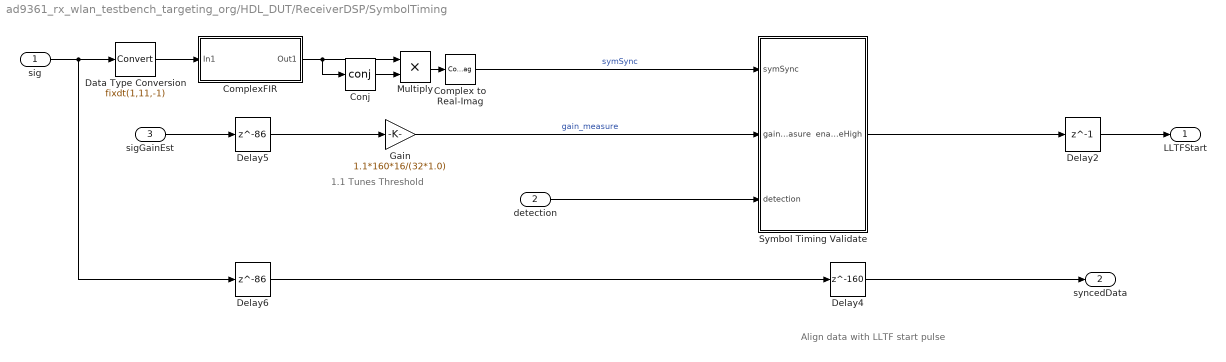
== system ad9361_rx_wlan_testbench_targeting_org/HDL_DUT/ReceiverDSP/SymbolTiming ==
  note: 1.1 Tunes Threshold
  note: Align data with LLTF start pulse
  sig : Inport  OutDataTypeStr=fixdt(1,11,-1)
  detection : Inport  Port=2
  sigGainEst : Inport  Port=3  OutDataTypeStr=fixdt(0,11,-12)
  Complex to Real-Imag : ComplexToRealImag  Output=Real
  ComplexFIR : Subsystem  mask{coefs=lltfFlip(1:80).'}
      mask prompts: coefs "Taps"
  Conj : Math  Operator=conj  OutDataTypeStr=double  SaturateOnIntegerOverflow=on
  Data Type Conversion : DataTypeConversion  OutDataTypeStr=fixdt(1,11,-1)
  Delay2 : Delay  DelayLength=1
  Delay4 : Delay  DelayLength=160
  Delay5 : Delay  DelayLength=86
  Delay6 : Delay  DelayLength=86
  Gain : Gain  Gain=1.1*160*16/(32*1.0)  ParamDataTypeStr=fixdt(0,11,4)  OutDataTypeStr=fixdt(0,11,-18)  SaturateOnIntegerOverflow=on
  Multiply : Product  OutDataTypeStr=fixdt(1,11,-21)
  Symbol Timing Validate : Subsystem
  LLTFStart : Outport  VectorParamsAs1DForOutWhenUnconnected=off
  syncedData : Outport  Port=2  OutDataTypeStr=fixdt(1,11,-1)  VectorParamsAs1DForOutWhenUnconnected=off
  wires:
  sigGainEst/1 -> Delay5/1
  Multiply/1 -> Complex to Real-Imag/1
  Delay2/1 -> LLTFStart/1
  Conj/1 -> Multiply/2
  sig/1 -> Data Type Conversion/1, Delay6/1
  Delay4/1 -> syncedData/1
  Delay5/1 -> Gain/1
  ComplexFIR/1(Out1) -> Multiply/1, Conj/1
  Data Type Conversion/1 -> ComplexFIR/1(In1)
  Delay6/1 -> Delay4/1
  Complex to Real-Imag/1 -> Symbol Timing Validate/1(symSync)  "symSync"
  Gain/1 -> Symbol Timing Validate/2(gain_measure)  "gain_measure"
  detection/1 -> Symbol Timing Validate/3(detection)
  Symbol Timing Validate/1(enableHigh) -> Delay2/1

== system ad9361_rx_wlan_testbench_targeting_org/HDL_DUT/ReceiverDSP/CFOCorrection/Average CFO Esimates ==
  note: Only take measurements when high for several cylces to help remote random burst
  In1 : Inport
  In2 : Inport  Port=2  OutDataTypeStr=fixdt(1,11,-10)
  AverageCFOEstimates1 : Subsystem  mask{N=15}
      mask prompts: N "Taps"
  Logical Operator : Logic  Inputs=1  AllPortsSameDT=off  OutDataTypeStr=boolean
  Tapped Delay : simulink/Discrete/Tapped Delay  vinit=0.0  samptime=-1  NumDelays=4  DelayOrder=Oldest  includeCurrent=off
  Out1 : Outport  VectorParamsAs1DForOutWhenUnconnected=off
  Out2 : Outport  Port=2  OutDataTypeStr=fixdt(1,11,-3)  VectorParamsAs1DForOutWhenUnconnected=off
  wires:
  Tapped Delay/1 -> Logical Operator/1
  AverageCFOEstimates1/1(Out1) -> Out2/1
  In2/1 -> AverageCFOEstimates1/1(In1)
  Logical Operator/1 -> Out1/1, AverageCFOEstimates1/Enable
  In1/1 -> Tapped Delay/1

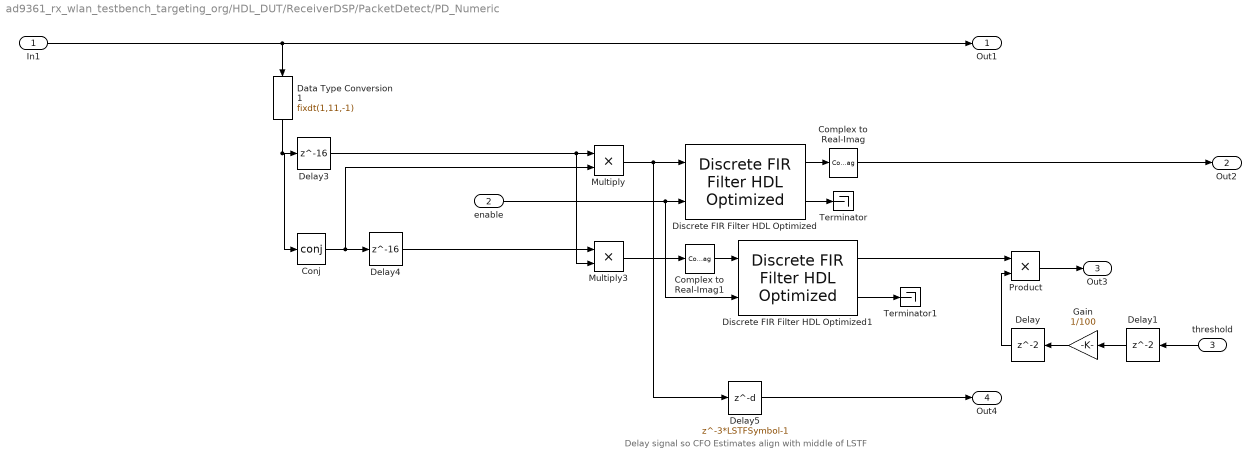
== system ad9361_rx_wlan_testbench_targeting_org/HDL_DUT/ReceiverDSP/PacketDetect/PD_Numeric ==
  note: Delay signal so CFO Estimates align with middle of LSTF
  In1 : Inport  OutDataTypeStr=fixdt(1,11,-1)
  enable : Inport  Port=2  OutDataTypeStr=boolean
  threshold : Inport  Port=3  OutDataTypeStr=fixdt(0,11,4)
  Complex to Real-Imag : ComplexToRealImag  Output=Real
  Complex to Real-Imag1 : ComplexToRealImag  Output=Real
  Conj : Math  Operator=conj  OutDataTypeStr=double  SaturateOnIntegerOverflow=on
  Data Type Conversion1 : DataTypeConversion  OutDataTypeStr=fixdt(1,11,-1)  SaturateOnIntegerOverflow=on
  Delay : Delay
  Delay1 : Delay
  Delay3 : Delay  DelayLength=16
  Delay4 : Delay  DelayLength=16
  Delay5 : Delay  DelayLength=3*LSTFSymbol-1
  Discrete FIR Filter HDL Optimized : dsphdlfiltering/Discrete FIR Filter HDL Optimized  NumeratorSource=Property  Numerator=ones(1,LSTFSymbol)  NumeratorPrototype=[ 0.5, 0.5 ]  FilterStructure=Direct form systolic  SerializationOption=Minimum number of cycles between valid input samples  NumberOfCycles=2  NumberOfMultipliers=2  SimulateUsing=Code generation  roundingMode=Floor  overflowMode=on  CoefficientsDataTypeStr=Inherit: Same word length as input  CoefficientsMin=[]  CoefficientsMax=[]  OutputDataTypeStr=Inherit: Same word length as input  OutputMin=[]  OutputMax=[]  ResetInputPort=off  HDLGlobalReset=off
      settings: SourceProductName=DSP System Toolbox  SourceProductBaseCode=DS
  Discrete FIR Filter HDL Optimized1 : dsphdlfiltering/Discrete FIR Filter HDL Optimized  NumeratorSource=Property  Numerator=ones(1,LSTFSymbol)  NumeratorPrototype=[ 0.5, 0.5 ]  FilterStructure=Direct form systolic  SerializationOption=Minimum number of cycles between valid input samples  NumberOfCycles=2  NumberOfMultipliers=2  SimulateUsing=Code generation  roundingMode=Floor  overflowMode=on  CoefficientsDataTypeStr=Inherit: Same word length as input  CoefficientsMin=[]  CoefficientsMax=[]  OutputDataTypeStr=Inherit: Same word length as input  OutputMin=[]  OutputMax=[]  ResetInputPort=off  HDLGlobalReset=off
      settings: SourceProductName=DSP System Toolbox  SourceProductBaseCode=DS
  Gain : Gain  Gain=1/100  ParamDataTypeStr=fixdt(0,11,17)  OutDataTypeStr=fixdt(0,11,11)
  Multiply : Product  OutDataTypeStr=fixdt(1,11,-11)  SaturateOnIntegerOverflow=on
  Multiply3 : Product  OutDataTypeStr=fixdt(1,11,-12)
  Product : Product  OutDataTypeStr=fixdt(0,11,-13)  SaturateOnIntegerOverflow=on
  Terminator : Terminator
  Terminator1 : Terminator
  Out1 : Outport  OutDataTypeStr=fixdt(1,11,-1)  VectorParamsAs1DForOutWhenUnconnected=off
  Out2 : Outport  Port=2  VectorParamsAs1DForOutWhenUnconnected=off
  Out3 : Outport  Port=3  OutDataTypeStr=fixdt(0,11,-13)  VectorParamsAs1DForOutWhenUnconnected=off
  Out4 : Outport  Port=4  OutDataTypeStr=fixdt(1,11,-11)  VectorParamsAs1DForOutWhenUnconnected=off
  wires:
  Delay4/1 -> Multiply3/1
  Discrete FIR Filter HDL Optimized1/2 -> Terminator1/1
  Conj/1 -> Multiply/2, Delay4/1
  Delay5/1 -> Out4/1
  Discrete FIR Filter HDL Optimized/1 -> Complex to Real-Imag/1
  enable/1 -> Discrete FIR Filter HDL Optimized1/2, Discrete FIR Filter HDL Optimized/2
  Multiply/1 -> Discrete FIR Filter HDL Optimized/1, Delay5/1
  Discrete FIR Filter HDL Optimized/2 -> Terminator/1
  Multiply3/1 -> Complex to Real-Imag1/1
  Complex to Real-Imag1/1 -> Discrete FIR Filter HDL Optimized1/1
  Product/1 -> Out3/1
  Discrete FIR Filter HDL Optimized1/1 -> Product/1
  Delay1/1 -> Gain/1
  Delay/1 -> Product/2
  Gain/1 -> Delay/1
  threshold/1 -> Delay1/1
  Delay3/1 -> Multiply3/2, Multiply/1
  In1/1 -> Out1/1, Data Type Conversion1/1
  Data Type Conversion1/1 -> Conj/1, Delay3/1
  Complex to Real-Imag/1 -> Out2/1

== system ad9361_rx_wlan_testbench_targeting_org/HDL_DUT/ReceiverDSP/PacketDetect/Subsystem ==
  In1 : Inport  OutDataTypeStr=fixdt(1,11,-13)
  In3 : Inport  Port=2  OutDataTypeStr=fixdt(0,11,-13)
  In4 : Inport  Port=3
  Compare To Constant : simulink/Logic and Bit Operations/Compare To Constant  relop=>=  const=2e6  OutDataTypeStr=boolean
  Enabled Subsystem : Subsystem  TreatAsAtomicUnit=on
  GreaterThan : RelationalOperator  Operator=>  OutDataTypeStr=boolean  RndMeth=Simplest
  Logical Operator : Logic  Inputs=3  AllPortsSameDT=off  OutDataTypeStr=boolean
  Logical Operator1 : Logic  Inputs=1  AllPortsSameDT=off  OutDataTypeStr=boolean
  Tapped Delay : simulink/Discrete/Tapped Delay  vinit=0.0  samptime=-1  NumDelays=32  DelayOrder=Oldest  includeCurrent=off
  detection : Outport  VectorParamsAs1DForOutWhenUnconnected=off
  Out2 : Outport  Port=2  OutDataTypeStr=fixdt(0,11,-12)  VectorParamsAs1DForOutWhenUnconnected=off
  wires:
  Logical Operator/1 -> Tapped Delay/1
  In4/1 -> Logical Operator/2
  In1/1 -> GreaterThan/1  "sigPath"
  Logical Operator1/1 -> detection/1, Enabled Subsystem/Enable  "pdCheck"
  Enabled Subsystem/1(Out1) -> Out2/1
  GreaterThan/1 -> Logical Operator/1
  In3/1 -> Compare To Constant/1, Enabled Subsystem/1(In1), GreaterThan/2  "powerPath"
  Tapped Delay/1 -> Logical Operator1/1
  Compare To Constant/1 -> Logical Operator/3

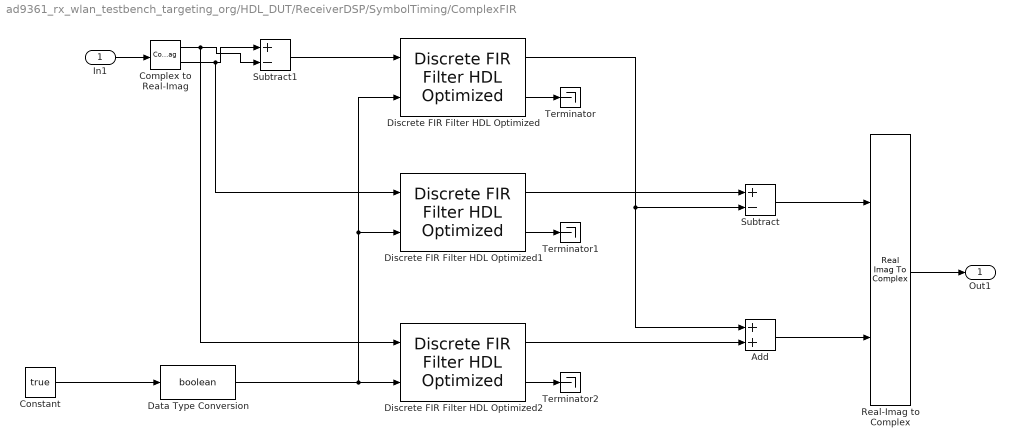
== system ad9361_rx_wlan_testbench_targeting_org/HDL_DUT/ReceiverDSP/SymbolTiming/ComplexFIR ==
  In1 : Inport  OutDataTypeStr=fixdt(1,11,-1)
  Add : Sum  AccumDataTypeStr=fixdt(1,11,-5)  OutDataTypeStr=fixdt(1,11,-5)
  Complex to Real-Imag : ComplexToRealImag
  Constant : Constant  Value=true  OutDataTypeStr=fixdt(0,11,10)  SampleTime=-1
  Data Type Conversion : DataTypeConversion  OutDataTypeStr=boolean
  Discrete FIR Filter HDL Optimized : dsphdlfiltering/Discrete FIR Filter HDL Optimized  NumeratorSource=Property  Numerator=real(coefs)  NumeratorPrototype=[ 0.5, 0.5 ]  FilterStructure=Direct form systolic  SerializationOption=Minimum number of cycles between valid input samples  NumberOfCycles=2  NumberOfMultipliers=2  SimulateUsing=Code generation  roundingMode=Floor  overflowMode=off  CoefficientsDataTypeStr=Inherit: Same word length as input  CoefficientsMin=[]  CoefficientsMax=[]  OutputMin=[]  OutputMax=[]  ResetInputPort=off  HDLGlobalReset=off
      settings: SourceProductName=DSP System Toolbox  SourceProductBaseCode=DS
  Discrete FIR Filter HDL Optimized1 : dsphdlfiltering/Discrete FIR Filter HDL Optimized  NumeratorSource=Property  Numerator=real(coefs)-imag(coefs)  NumeratorPrototype=[ 0.5, 0.5 ]  FilterStructure=Direct form systolic  SerializationOption=Minimum number of cycles between valid input samples  NumberOfCycles=2  NumberOfMultipliers=2  SimulateUsing=Code generation  roundingMode=Floor  overflowMode=off  CoefficientsDataTypeStr=Inherit: Same word length as input  CoefficientsMin=[]  CoefficientsMax=[]  OutputMin=[]  OutputMax=[]  ResetInputPort=off  HDLGlobalReset=off
      settings: SourceProductName=DSP System Toolbox  SourceProductBaseCode=DS
  Discrete FIR Filter HDL Optimized2 : dsphdlfiltering/Discrete FIR Filter HDL Optimized  NumeratorSource=Property  Numerator=real(coefs)+imag(coefs)  NumeratorPrototype=[ 0.5, 0.5 ]  FilterStructure=Direct form systolic  SerializationOption=Minimum number of cycles between valid input samples  NumberOfCycles=2  NumberOfMultipliers=2  SimulateUsing=Code generation  roundingMode=Floor  overflowMode=off  CoefficientsDataTypeStr=Inherit: Same word length as input  CoefficientsMin=[]  CoefficientsMax=[]  OutputMin=[]  OutputMax=[]  ResetInputPort=off  HDLGlobalReset=off
      settings: SourceProductName=DSP System Toolbox  SourceProductBaseCode=DS
  Real-Imag to Complex : RealImagToComplex
  Subtract : Sum  Inputs=+-  AccumDataTypeStr=fixdt(1,11,-5)  OutDataTypeStr=fixdt(1,11,-5)
  Subtract1 : Sum  Inputs=+-  AccumDataTypeStr=fixdt(1,11,-1)  OutDataTypeStr=fixdt(1,11,-1)
  Terminator : Terminator
  Terminator1 : Terminator
  Terminator2 : Terminator
  Out1 : Outport  OutDataTypeStr=fixdt(1,11,-5)  VectorParamsAs1DForOutWhenUnconnected=off
  wires:
  Discrete FIR Filter HDL Optimized1/1 -> Subtract/1
  Discrete FIR Filter HDL Optimized/1 -> Add/1, Subtract/2
  Discrete FIR Filter HDL Optimized2/1 -> Add/2
  Subtract/1 -> Real-Imag to Complex/1
  Add/1 -> Real-Imag to Complex/2
  Real-Imag to Complex/1 -> Out1/1
  In1/1 -> Complex to Real-Imag/1
  Subtract1/1 -> Discrete FIR Filter HDL Optimized/1
  Complex to Real-Imag/2 -> Discrete FIR Filter HDL Optimized1/1, Subtract1/1
  Complex to Real-Imag/1 -> Discrete FIR Filter HDL Optimized2/1, Subtract1/2
  Discrete FIR Filter HDL Optimized/2 -> Terminator/1
  Discrete FIR Filter HDL Optimized1/2 -> Terminator1/1
  Discrete FIR Filter HDL Optimized2/2 -> Terminator2/1
  Constant/1 -> Data Type Conversion/1
  Data Type Conversion/1 -> Discrete FIR Filter HDL Optimized1/2, Discrete FIR Filter HDL Optimized/2, Discrete FIR Filter HDL Optimized2/2

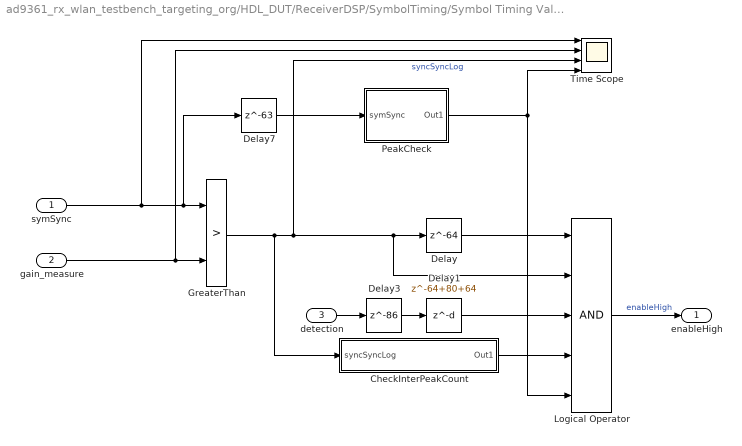
== system ad9361_rx_wlan_testbench_targeting_org/HDL_DUT/ReceiverDSP/SymbolTiming/Symbol Timing Validate ==
  symSync : Inport
  gain_measure : Inport  Port=2
  detection : Inport  Port=3
  CheckInterPeakCount : Subsystem
  Delay : Delay  DelayLength=64
  Delay1 : Delay  DelayLength=64+80+64
  Delay3 : Delay  DelayLength=86
  Delay7 : Delay  DelayLength=63
  GreaterThan : RelationalOperator  Operator=>  OutDataTypeStr=boolean  RndMeth=Simplest
  Logical Operator : Logic  Inputs=5  AllPortsSameDT=off  OutDataTypeStr=boolean
  PeakCheck : Subsystem
  Time Scope : Scope  NumInputPorts=4
  enableHigh : Outport  VectorParamsAs1DForOutWhenUnconnected=off
  wires:
  Delay3/1 -> Delay1/1
  gain_measure/1 -> Time Scope/2, GreaterThan/2
  Logical Operator/1 -> enableHigh/1  "enableHigh"
  CheckInterPeakCount/1(Out1) -> Logical Operator/4
  GreaterThan/1 -> CheckInterPeakCount/1(syncSyncLog), Time Scope/3, Logical Operator/2, Delay/1  "syncSyncLog"
  Delay/1 -> Logical Operator/1
  symSync/1 -> Time Scope/1, Delay7/1, GreaterThan/1
  Delay7/1 -> PeakCheck/1(symSync)
  PeakCheck/1(Out1) -> Time Scope/4, Logical Operator/5
  detection/1 -> Delay3/1
  Delay1/1 -> Logical Operator/3

== system ad9361_rx_wlan_testbench_targeting_org/HDL_DUT/ReceiverDSP/CFOCorrection/Average CFO Esimates/AverageCFOEstimates1 ==
  In1 : Inport  OutDataTypeStr=fixdt(1,11,-10)
  Enable : EnablePort
  Delay2 : Delay  DelayLength=1
  Gain : Gain  Gain=1/N  ParamDataTypeStr=fixdt(0,11,14)  OutDataTypeStr=fixdt(1,11,-3)
  Sum of Elements : Sum  Inputs=+  AccumDataTypeStr=fixdt(1,11,-7)  OutDataTypeStr=fixdt(1,11,-7)
  Tapped Delay : simulink/Discrete/Tapped Delay  vinit=0.0  samptime=-1  NumDelays=N  DelayOrder=Oldest  includeCurrent=off
  Out1 : Outport  OutDataTypeStr=fixdt(1,11,-3)  InitialOutput=0  VectorParamsAs1DForOutWhenUnconnected=off
  wires:
  Tapped Delay/1 -> Sum of Elements/1
  In1/1 -> Tapped Delay/1
  Sum of Elements/1 -> Delay2/1
  Gain/1 -> Out1/1
  Delay2/1 -> Gain/1

== system ad9361_rx_wlan_testbench_targeting_org/HDL_DUT/ReceiverDSP/PacketDetect/Subsystem/Enabled Subsystem ==
  In1 : Inport  OutDataTypeStr=fixdt(0,11,-13)
  Enable : EnablePort
  Delay2 : Delay  DelayLength=1
  Gain : Gain  Gain=1/15  ParamDataTypeStr=fixdt(0,11,14)  OutDataTypeStr=fixdt(0,11,-12)
  Sum of Elements : Sum  Inputs=+  AccumDataTypeStr=fixdt(0,11,-16)  OutDataTypeStr=fixdt(0,11,-16)
  Tapped Delay : simulink/Discrete/Tapped Delay  vinit=0.0  samptime=-1  NumDelays=15  DelayOrder=Oldest  includeCurrent=off
  Out1 : Outport  OutDataTypeStr=fixdt(0,11,-12)  InitialOutput=0  VectorParamsAs1DForOutWhenUnconnected=off
  wires:
  In1/1 -> Tapped Delay/1
  Tapped Delay/1 -> Sum of Elements/1
  Sum of Elements/1 -> Delay2/1
  Gain/1 -> Out1/1
  Delay2/1 -> Gain/1

== system ad9361_rx_wlan_testbench_targeting_org/HDL_DUT/ReceiverDSP/SymbolTiming/Symbol Timing Validate/CheckInterPeakCount ==
  note: Allowed Peaks
  note: Window
  note: Offset From Front Peak
  syncSyncLog : Inport
  Compare To Constant : simulink/Logic and Bit Operations/Compare To Constant  relop=<=  const=2  OutDataTypeStr=boolean
  Delay : Delay  DelayLength=15
  Delay7 : Delay  DelayLength=1
  Sum of Elements : Sum  Inputs=+
  Tapped Delay : simulink/Discrete/Tapped Delay  vinit=0.0  samptime=-1  NumDelays=30  DelayOrder=Oldest  includeCurrent=off
  Out1 : Outport  VectorParamsAs1DForOutWhenUnconnected=off
  wires:
  Sum of Elements/1 -> Compare To Constant/1
  Delay/1 -> Tapped Delay/1
  syncSyncLog/1 -> Delay/1
  Delay7/1 -> Sum of Elements/1
  Compare To Constant/1 -> Out1/1
  Tapped Delay/1 -> Delay7/1
